simulink model "SF004B_AssiSumLim"  (R2013b)
settings: Solver=FixedStepDiscrete  StartTime=0.0  StopTime=1  FixedStep=.002  RelTol=1e-3
values from neighbouring files (symbols this model uses):
  AssiSumLimNtc0x0C4FailStep = DataDict.Calibration    [SF004B_AssiSumLim_DataDict.m]
  AssiSumLimNtc0x0C4PassStep = DataDict.Calibration    [SF004B_AssiSumLim_DataDict.m]
  AssiSumLimPullCmpLim = DataDict.Calibration    [SF004B_AssiSumLim_DataDict.m]
  CMDTHD_MOTNWTMTR_F32 = DataDict.Constant    [SF004B_AssiSumLim_DataDict.m]
  E_NOT_OK = DataDict.Constant    [AR200A_ArSuprt_DataDict.m]
  E_OK = DataDict.Constant    [AR200A_ArSuprt_DataDict.m]
  MOTTQZERO_MOTNWTMTR_F32 = DataDict.Constant    [SF004B_AssiSumLim_DataDict.m]
  VEHSPDTHD_KPH_F32 = DataDict.Constant    [SF004B_AssiSumLim_DataDict.m]
undefined symbols (not defined in the file or in its folder): NtcNr1, NtcSts1, SigQlfr1
libraries: simulink x11, NexteerUtilities x7, NxtrSign x1, NxtrAbslt x1
(part 2 of 3)

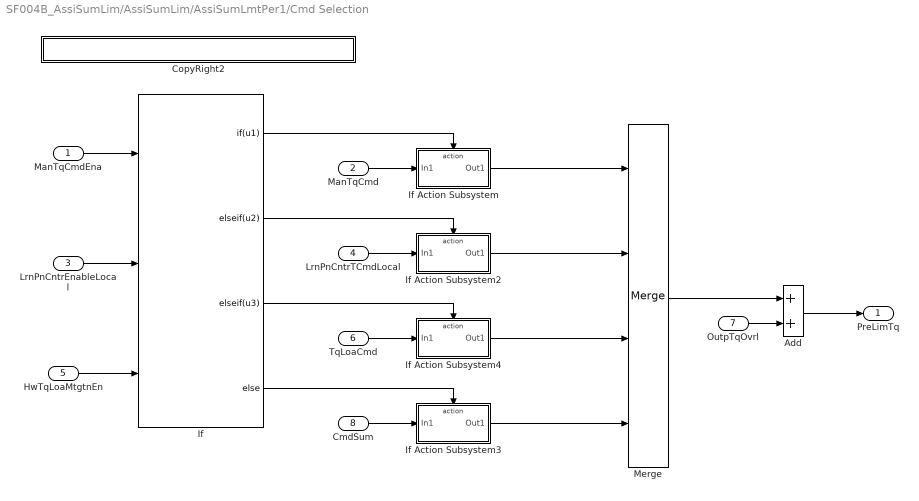
== system SF004B_AssiSumLim/AssiSumLim/AssiSumLmtPer1/Cmd Selection ==
  ManTqCmdEna : Inport  OutDataTypeStr=boolean  PortDimensions=1
  ManTqCmd : Inport  RequirementInfo="{'linktype_rmi_doors' '00007fee (/E-STEER Core/SubSystem Specifications/Application Functions/SF004B Assist Summation and Limiting- Current)' '#SF004B_259' 'true' 'REQ:  SF004B_259' '' } %GIDa_6d4687b5_3845_4db2_a601_45ef4cdee017"  Port=2  PortDimensions=1
  LrnPnCntrEnableLocal : Inport  Port=3  PortDimensions=1
  LrnPnCntrTCmdLocal : Inport  RequirementInfo="{'linktype_rmi_doors' '00007fee (/E-STEER Core/SubSystem Specifications/Application Functions/SF004B Assist Summation and Limiting- Current)' '#SF004B_259' 'true' 'REQ:  SF004B_259' '' } %GIDa_5a22f24a_6e36_40a7_96fa_9b9f9ce3bdd4"  Port=4  PortDimensions=1
  HwTqLoaMtgtnEn : Inport  Port=5  PortDimensions=1
  TqLoaCmd : Inport  RequirementInfo="{'linktype_rmi_doors' '00007fee (/E-STEER Core/SubSystem Specifications/Application Functions/SF004B Assist Summation and Limiting- Current)' '#SF004B_259' 'true' 'REQ:  SF004B_259' '' } %GIDa_d1377691_6c28_435b_bb8c_3dc15aacdf96"  Port=6  PortDimensions=1
  OutpTqOvrl : Inport  RequirementInfo="{'linktype_rmi_doors' '00007fee (/E-STEER Core/SubSystem Specifications/Application Functions/SF004B Assist Summation and Limiting- Current)' '#SF004B_262' 'true' 'REQ:  SF004B_262' '' } %GIDa_e8533355_9a04_466e_861e_ebd78117bea2"  Port=7
  CmdSum : Inport  RequirementInfo="{'linktype_rmi_doors' '00007fee (/E-STEER Core/SubSystem Specifications/Application Functions/SF004B Assist Summation and Limiting- Current)' '#SF004B_259' 'true' 'REQ:  SF004B_259' '' } %GIDa_7c3c2e40_c5fa_4ce2_b662_add04edc3132"  Port=8
  Add : Sum  RequirementInfo="{'linktype_rmi_doors' '00007fee (/E-STEER Core/SubSystem Specifications/Application Functions/SF004B Assist Summation and Limiting- Current)' '#SF004B_262' 'true' 'REQ:  SF004B_262' '' } %GIDa_34ce2345_5df1_4df2_a470_66ac93518d9f"
  CopyRight2 : Subsystem  Description=|  mask(Copyright Information){none=on}
      | Copyright info block.                                               
      |                                                                     
      | Place copyright information at the top of every subsystem in design.
      mask prompts: none "No parameters"
      mask help: Place copyright information at the top of every subsystem in design.
      mask Display:
      | NxtrConf = 'Nexteer Confidential';
      | 
      | sys = bdroot; %handle for the current model ("system")
      | first = get_param(sys,'Created');
      | first = first(end-3:end);  %year is last four digits
      | 
      | last = get_param(sys,'LastModifiedDate');
      | if isempty(last)
      |     last = datestr(now,'yyyy');
      | else
      |     last = last(end-3:end);
      | end
      | 
      | if strcmp(first,last)
      |     fprintf('%s -- Copyright %s Nexteer',NxtrConf,first)
      | else
      |     fprintf('%s -- %s%s- %s Nexteer',NxtrConf,char(169),first,last)
      | end
  If : If  RequirementInfo="{'linktype_rmi_doors' '00007fee (/E-STEER Core/SubSystem Specifications/Application Functions/SF004B Assist Summation and Limiting- Current)' '#SF004B_219' 'true' 'REQ:  SF004B_219' '' } %GIDa_35ee30c3_2e73_4baf_af04_8a15c809cf7f"  NumInputs=3  IfExpression=u1  ElseIfExpressions=u2, u3
  If Action Subsystem : Subsystem  TreatAsAtomicUnit=on
      settings: RTWSystemCode=Inline
  If Action Subsystem2 : Subsystem  TreatAsAtomicUnit=on
      settings: RTWSystemCode=Inline
  If Action Subsystem3 : Subsystem  TreatAsAtomicUnit=on
      settings: RTWSystemCode=Inline
  If Action Subsystem4 : Subsystem  TreatAsAtomicUnit=on
      settings: RTWSystemCode=Inline
  Merge : Merge  Inputs=4
  PreLimTq : Outport
  wires:
  Merge/1 -> Add/1
  ManTqCmd/1 -> If Action Subsystem/1(In1)
  LrnPnCntrTCmdLocal/1 -> If Action Subsystem2/1(In1)
  TqLoaCmd/1 -> If Action Subsystem4/1(In1)
  CmdSum/1 -> If Action Subsystem3/1(In1)
  If/1 -> If Action Subsystem/Action
  If/2 -> If Action Subsystem2/Action
  If/3 -> If Action Subsystem4/Action
  If/4 -> If Action Subsystem3/Action
  ManTqCmdEna/1 -> If/1
  LrnPnCntrEnableLocal/1 -> If/2
  HwTqLoaMtgtnEn/1 -> If/3
  If Action Subsystem2/1(Out1) -> Merge/2
  If Action Subsystem/1(Out1) -> Merge/1
  If Action Subsystem4/1(Out1) -> Merge/3
  If Action Subsystem3/1(Out1) -> Merge/4
  OutpTqOvrl/1 -> Add/2
  Add/1 -> PreLimTq/1

== system SF004B_AssiSumLim/AssiSumLim/AssiSumLmtPer1/Cmd Summation ==
  AssiCmd : Inport  PortDimensions=1
  EotAssiSca : Inport  Port=2  PortDimensions=1
  LimdRtn : Inport  Port=3  PortDimensions=1
  CombdDampg : Inport  Port=4  PortDimensions=1
  AssisEotDampg : Inport  Port=5  PortDimensions=1
  WhlImbRejctnCmd : Inport  Port=6  PortDimensions=1
  PullCmpCmd : Inport  RequirementInfo={} %GIDa_3c33220d_3b7c_4bff_a881_a0220ab0f687  Port=7
  TqSteerMtgtnCmd : Inport  RequirementInfo={} %GIDa_a55a9c38_6f5b_4402_afc7_80609bbfcfbd  Port=8
  EotActvCmd : Inport  Port=9  PortDimensions=1
  CopyRight2 : Subsystem  Description=|  mask(Copyright Information){none=on}
      | Copyright info block.                                               
      |                                                                     
      | Place copyright information at the top of every subsystem in design.
      mask prompts: none "No parameters"
      mask help: Place copyright information at the top of every subsystem in design.
      mask Display:
      | NxtrConf = 'Nexteer Confidential';
      | 
      | sys = bdroot; %handle for the current model ("system")
      | first = get_param(sys,'Created');
      | first = first(end-3:end);  %year is last four digits
      | 
      | last = get_param(sys,'LastModifiedDate');
      | if isempty(last)
      |     last = datestr(now,'yyyy');
      | else
      |     last = last(end-3:end);
      | end
      | 
      | if strcmp(first,last)
      |     fprintf('%s -- Copyright %s Nexteer',NxtrConf,first)
      | else
      |     fprintf('%s -- %s%s- %s Nexteer',NxtrConf,char(169),first,last)
      | end
  Product : Product  RequirementInfo="{'linktype_rmi_doors' '00007fee (/E-STEER Core/SubSystem Specifications/Application Functions/SF004B Assist Summation and Limiting- Current)' '#SF004B_213' 'true' 'REQ:  SF004B_213' '' } %GIDa_54f00f48_10ff_4ca6_98ab_f17879de9b5f"  RndMeth=Zero
  Summation : Sum  RequirementInfo="{'linktype_rmi_doors' '00007fee (/E-STEER Core/SubSystem Specifications/Application Functions/SF004B Assist Summation and Limiting- Current)' '#SF004B_216' 'true' 'REQ:  SF004B_216' '' } %GIDa_b057e6a3_dc30_4611_b70e_8624ca67ab72"  Inputs=+---++++
  CmdSum : Outport
  wires:
  Summation/1 -> CmdSum/1
  EotAssiSca/1 -> Product/2
  AssiCmd/1 -> Product/1
  CombdDampg/1 -> Summation/3
  LimdRtn/1 -> Summation/2
  Product/1 -> Summation/1  "ScaldAssiCmd"
  AssisEotDampg/1 -> Summation/4
  WhlImbRejctnCmd/1 -> Summation/5
  TqSteerMtgtnCmd/1 -> Summation/6
  EotActvCmd/1 -> Summation/8
  PullCmpCmd/1 -> Summation/7

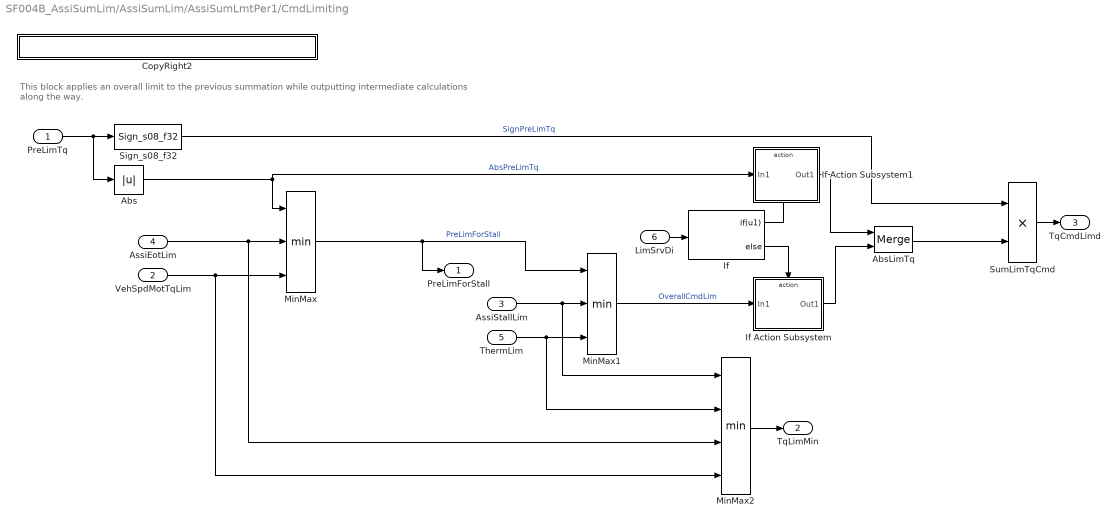
== system SF004B_AssiSumLim/AssiSumLim/AssiSumLmtPer1/CmdLimiting ==
  note: This block applies an overall limit to the previous summation while outputting intermediate calculations along the way.
  PreLimTq : Inport
  VehSpdMotTqLim : Inport  Port=2
  AssiStallLim : Inport  Port=3
  AssiEotLim : Inport  Port=4
  ThermLim : Inport  Port=5
  LimSrvDi : Inport  RequirementInfo={} %GIDa_99432472_4a71_4873_a7a5_b3a83e1be238  Port=6
  Abs : Abs
  AbsLimTq : Merge
  CopyRight2 : Subsystem  Description=|  mask(Copyright Information){none=on}
      | Copyright info block.                                               
      |                                                                     
      | Place copyright information at the top of every subsystem in design.
      mask prompts: none "No parameters"
      mask help: Place copyright information at the top of every subsystem in design.
      mask Display:
      | NxtrConf = 'Nexteer Confidential';
      | 
      | sys = bdroot; %handle for the current model ("system")
      | first = get_param(sys,'Created');
      | first = first(end-3:end);  %year is last four digits
      | 
      | last = get_param(sys,'LastModifiedDate');
      | if isempty(last)
      |     last = datestr(now,'yyyy');
      | else
      |     last = last(end-3:end);
      | end
      | 
      | if strcmp(first,last)
      |     fprintf('%s -- Copyright %s Nexteer',NxtrConf,first)
      | else
      |     fprintf('%s -- %s%s- %s Nexteer',NxtrConf,char(169),first,last)
      | end
  If : If  RequirementInfo="{'linktype_rmi_doors' '00007fee (/E-STEER Core/SubSystem Specifications/Application Functions/SF004B Assist Summation and Limiting- Current)' '#SF004B_274' 'true' 'REQ:  SF004B_274' '' ; 'linktype_rmi_doors' '00007fee (/E-STEER Core/SubSystem Specifications/Application Functions/SF004B Assist Summation and Limiting- Current)' '#SF004B_231' 'true' 'REQ:  SF004B_231' '' } %GIDa_b6ca4058_5217_4cfe_92e9_f2747dcd1412"  IfExpression=u1
  If Action Subsystem : Subsystem  TreatAsAtomicUnit=on
  If Action Subsystem1 : Subsystem  TreatAsAtomicUnit=on
  MinMax : MinMax  RequirementInfo="{'linktype_rmi_doors' '00007fee (/E-STEER Core/SubSystem Specifications/Application Functions/SF004B Assist Summation and Limiting- Current)' '#SF004B_233' 'true' 'REQ:  SF004B_233' '' } %GIDa_b7889423_6edb_4d87_96b6_21fb77770748"  Inputs=3
  MinMax1 : MinMax  RequirementInfo="{'linktype_rmi_doors' '00007fee (/E-STEER Core/SubSystem Specifications/Application Functions/SF004B Assist Summation and Limiting- Current)' '#SF004B_232' 'true' 'REQ:  SF004B_232' '' } %GIDa_f7d227db_8738_4fd0_b4dd_de7410152b8b"  Inputs=3
  MinMax2 : MinMax  RequirementInfo="{'linktype_rmi_doors' '00007fee (/E-STEER Core/SubSystem Specifications/Application Functions/SF004B Assist Summation and Limiting- Current)' '#SF004B_234' 'true' 'REQ:  SF004B_234' '' } %GIDa_87d08d71_c97c_4c6d_9ff2_320bb954175b"  Inputs=4
  Sign_s08_f32 : NxtrSign/Sign_s08_f32  SFunctionSpec=int8 y1 = Sign_s08_f32(single u1)
  SumLimTqCmd : Product  RequirementInfo={} %GIDa_2c601304_2811_4536_8544_69d3b3eae512  RndMeth=Zero
  PreLimForStall : Outport
  TqLimMin : Outport  Port=2
  TqCmdLimd : Outport  Port=3
  wires:
  PreLimTq/1 -> Abs/1, Sign_s08_f32/1
  AssiEotLim/1 -> MinMax2/3, MinMax/2
  Abs/1 -> If Action Subsystem1/1(In1), MinMax/1  "AbsPreLimTq"
  MinMax1/1 -> If Action Subsystem/1(In1)  "OverallCmdLim"
  LimSrvDi/1 -> If/1
  VehSpdMotTqLim/1 -> MinMax2/4, MinMax/3
  AssiStallLim/1 -> MinMax2/1, MinMax1/2
  ThermLim/1 -> MinMax2/2, MinMax1/3
  MinMax/1 -> MinMax1/1, PreLimForStall/1  "PreLimForStall"
  AbsLimTq/1 -> SumLimTqCmd/2
  Sign_s08_f32/1 -> SumLimTqCmd/1  "SignPreLimTq"
  SumLimTqCmd/1 -> TqCmdLimd/1
  MinMax2/1 -> TqLimMin/1
  If/1 -> If Action Subsystem1/Action
  If/2 -> If Action Subsystem/Action
  If Action Subsystem1/1(Out1) -> AbsLimTq/1
  If Action Subsystem/1(Out1) -> AbsLimTq/2

== system SF004B_AssiSumLim/AssiSumLim/AssiSumLmtPer1/CopyRight2 ==

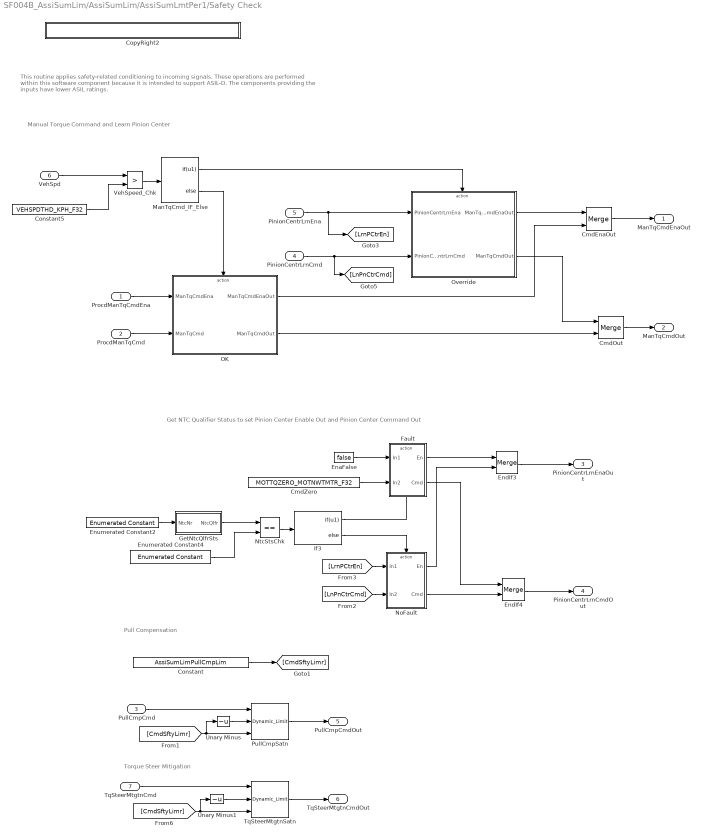
== system SF004B_AssiSumLim/AssiSumLim/AssiSumLmtPer1/Safety Check ==
  note: Get NTC Qualifier Status to set Pinion Center Enable Out and Pinion Center Command Out
  note: This routine applies safety-related conditioning to incoming signals.  These operations are performed within this software component
      | because it is intended to support ASIL-D.  The components providing the inputs have lower ASIL ratings.
  note: Pull Compensation
  note: Manual Torque Command and Learn Pinion Center
  note: Torque Steer Mitigation
  ProcdManTqCmdEna : Inport  OutDataTypeStr=boolean  PortDimensions=1
  ProcdManTqCmd : Inport  Port=2  PortDimensions=1
  PullCmpCmd : Inport  Port=3  PortDimensions=1
  PinionCentrLrnCmd : Inport  Port=4  PortDimensions=1
  PinionCentrLrnEna : Inport  Port=5  PortDimensions=1
  VehSpd : Inport  RequirementInfo="{'linktype_rmi_doors' '00007fee (/E-STEER Core/SubSystem Specifications/Application Functions/SF004B Assist Summation and Limiting- Current)' '#SF004B_290' 'true' 'REQ:  SF004B_290' '' ; 'linktype_rmi_doors' '00007fee (/E-STEER Core/SubSystem Specifications/Application Functions/SF004B Assist Summation and Limiting- Current)' '#SF004B_291' 'true' 'REQ:  SF004B_291' '' } %GIDa_9e2345ee_1316_4978_91a9_3c7026d77478"  Port=6  PortDimensions=1
  TqSteerMtgtnCmd : Inport  Port=7  PortDimensions=1
  CmdEnaOut : Merge
  CmdOut : Merge
  CmdZero : Constant  RequirementInfo="{'linktype_rmi_doors' '00007fee (/E-STEER Core/SubSystem Specifications/Application Functions/SF004B Assist Summation and Limiting- Current)' '#SF004B_273' 'true' 'REQ:  SF004B_273' '' } %GIDa_72c80312_63d9_41e1_a105_02d9b74c32c9"  Value=MOTTQZERO_MOTNWTMTR_F32
  Constant : Constant  RequirementInfo="{'linktype_rmi_doors' '00007fee (/E-STEER Core/SubSystem Specifications/Application Functions/SF004B Assist Summation and Limiting- Current)' '#SF004B_212' 'true' 'REQ:  SF004B_212' '' ; 'linktype_rmi_doors' '00007fee (/E-STEER Core/SubSystem Specifications/Application Functions/SF004B Assist Summation and Limiting- Current)' '#SF004B_296' 'true' 'REQ:  SF004B_296' '' } %GIDa_3116ad40_ee56_4034_a9ad_0e11ebed5c7d"  Value=AssiSumLimPullCmpLim
  Constant5 : Constant  RequirementInfo="{'linktype_rmi_doors' '00007fee (/E-STEER Core/SubSystem Specifications/Application Functions/SF004B Assist Summation and Limiting- Current)' '#SF004B_290' 'true' 'REQ:  SF004B_290' '' ; 'linktype_rmi_doors' '00007fee (/E-STEER Core/SubSystem Specifications/Application Functions/SF004B Assist Summation and Limiting- Current)' '#SF004B_291' 'true' 'REQ:  SF004B_291' '' } %GIDa_d7f1dc31_adb8_4977_a360_33e586f4483f"  Value=VEHSPDTHD_KPH_F32
  CopyRight2 : Subsystem  Description=|  mask(Copyright Information){none=on}
      | Copyright info block.                                               
      |                                                                     
      | Place copyright information at the top of every subsystem in design.
      mask prompts: none "No parameters"
      mask help: Place copyright information at the top of every subsystem in design.
      mask Display:
      | NxtrConf = 'Nexteer Confidential';
      | 
      | sys = bdroot; %handle for the current model ("system")
      | first = get_param(sys,'Created');
      | first = first(end-3:end);  %year is last four digits
      | 
      | last = get_param(sys,'LastModifiedDate');
      | if isempty(last)
      |     last = datestr(now,'yyyy');
      | else
      |     last = last(end-3:end);
      | end
      | 
      | if strcmp(first,last)
      |     fprintf('%s -- Copyright %s Nexteer',NxtrConf,first)
      | else
      |     fprintf('%s -- %s%s- %s Nexteer',NxtrConf,char(169),first,last)
      | end
  EnaFalse : Constant  RequirementInfo="{'linktype_rmi_doors' '00007fee (/E-STEER Core/SubSystem Specifications/Application Functions/SF004B Assist Summation and Limiting- Current)' '#SF004B_272' 'true' 'REQ:  SF004B_272' '' } %GIDa_5ff0557c_fca9_4b53_a4d3_a49375b62df5"  Value=false  OutDataTypeStr=boolean
  EndIf3 : Merge
  EndIf4 : Merge
  Enumerated Constant2 : simulink/Sources/Enumerated Constant  RequirementInfo="{'linktype_rmi_doors' '00007fee (/E-STEER Core/SubSystem Specifications/Application Functions/SF004B Assist Summation and Limiting- Current)' '#SF004B_270' 'true' 'REQ:  SF004B_270' '' } %GIDa_fe97f3de_4aa7_4587_b943_1a0b68072b4c"  OutDataTypeStr=Enum: NtcNr1  Value=NtcNr1.NTCNR_0X0C4  SampleTime=inf
  Enumerated Constant4 : simulink/Sources/Enumerated Constant  RequirementInfo="{'linktype_rmi_doors' '00007fee (/E-STEER Core/SubSystem Specifications/Application Functions/SF004B Assist Summation and Limiting- Current)' '#SF004B_270' 'true' 'REQ:  SF004B_270' '' } %GIDa_63663681_ffa3_4a91_a470_a2544b7c0835"  OutDataTypeStr=Enum: SigQlfr1  Value=SigQlfr1.SIGQLFR_FAILD  SampleTime=inf
  Fault : Subsystem  RequirementInfo="{'linktype_rmi_doors' '00007fee (/E-STEER Core/SubSystem Specifications/Application Functions/SF004B Assist Summation and Limiting- Current)' '#SF004B_270' 'true' 'REQ:  SF004B_270' '' } %GIDa_a6ae2e68_5cf5_45c1_b47e_16fabd600c68"  TreatAsAtomicUnit=on
      settings: RTWSystemCode=Inline
  GetNtcQlfrSts : Subsystem  RequirementInfo="{'linktype_rmi_doors' '00007fee (/E-STEER Core/SubSystem Specifications/Application Functions/SF004B Assist Summation and Limiting- Current)' '#SF004B_270' 'true' 'REQ:  SF004B_270' '' } %GIDa_160041d5_3f9d_403a_ac84_d13c70ea3b97"  TreatAsAtomicUnit=on  mask(GetNTC){}
      mask help: GetNTC library block
      settings: RTWSystemCode=Inline
  If3 : If  RequirementInfo="{'linktype_rmi_doors' '00007fee (/E-STEER Core/SubSystem Specifications/Application Functions/SF004B Assist Summation and Limiting- Current)' '#SF004B_270' 'true' 'REQ:  SF004B_270' '' } %GIDa_dbf14775_42f2_44d6_bdcc_28cea20182c7"  IfExpression=u1
  ManTqCmd_IF_Else : If  RequirementInfo="{'linktype_rmi_doors' '00007fee (/E-STEER Core/SubSystem Specifications/Application Functions/SF004B Assist Summation and Limiting- Current)' '#SF004B_290' 'true' 'REQ:  SF004B_290' '' ; 'linktype_rmi_doors' '00007fee (/E-STEER Core/SubSystem Specifications/Application Functions/SF004B Assist Summation and Limiting- Current)' '#SF004B_291' 'true' 'REQ:  SF004B_291' '' } %GIDa_5ecbdf41_6b0b_44e6_abca_066fe4f2cb92"  IfExpression=u1
  NoFault : Subsystem  TreatAsAtomicUnit=on
      settings: RTWSystemCode=Inline
  NtcStsChk : RelationalOperator  RequirementInfo="{'linktype_rmi_doors' '00007fee (/E-STEER Core/SubSystem Specifications/Application Functions/SF004B Assist Summation and Limiting- Current)' '#SF004B_270' 'true' 'REQ:  SF004B_270' '' } %GIDa_0dad4e9e_7eac_4b84_8c05_cc315494a582"  Operator===  OutDataTypeStr=boolean
  OK : Subsystem  TreatAsAtomicUnit=on
      settings: RTWSystemCode=Inline
  Override : Subsystem  RequirementInfo="{}  %GIDa_68c2586b_0b52_4b35_9c36_d935d27471ff"  TreatAsAtomicUnit=on
      settings: RTWSystemCode=Inline
  PullCmpSatn : NexteerUtilities/Dynamic_Limit  RequirementInfo="{'linktype_rmi_doors' '00007fee (/E-STEER Core/SubSystem Specifications/Application Functions/SF004B Assist Summation and Limiting- Current)' '#SF004B_212' 'true' 'REQ:  SF004B_212' '' } %GIDa_833cf9fb_40c9_409d_b2cf_b906ba45bd8b"
  TqSteerMtgtnSatn : NexteerUtilities/Dynamic_Limit  RequirementInfo="{'linktype_rmi_doors' '00007fee (/E-STEER Core/SubSystem Specifications/Application Functions/SF004B Assist Summation and Limiting- Current)' '#SF004B_296' 'true' 'REQ:  SF004B_296' '' } %GIDa_ee85d5d2_228e_4ce6_90fb_edd95af945f9"
  Unary Minus : UnaryMinus
  Unary Minus1 : UnaryMinus
  VehSpeed_Chk : RelationalOperator  RequirementInfo="{'linktype_rmi_doors' '00007fee (/E-STEER Core/SubSystem Specifications/Application Functions/SF004B Assist Summation and Limiting- Current)' '#SF004B_290' 'true' 'REQ:  SF004B_290' '' ; 'linktype_rmi_doors' '00007fee (/E-STEER Core/SubSystem Specifications/Application Functions/SF004B Assist Summation and Limiting- Current)' '#SF004B_291' 'true' 'REQ:  SF004B_291' '' } %GIDa_a6ce3cb5_8aa4_4683_a921_a710aa676490"  Operator=>  OutDataTypeStr=boolean
  ManTqCmdEnaOut : Outport
  ManTqCmdOut : Outport  Port=2
  PinionCentrLrnEnaOut : Outport  Port=3
  PinionCentrLrnCmdOut : Outport  Port=4
  PullCmpCmdOut : Outport  Port=5
  TqSteerMtgtnCmdOut : Outport  Port=6
  wires:
  PullCmpCmd/1 -> PullCmpSatn/1
  [CmdSftyLimr] -> Unary Minus/1, PullCmpSatn/3
  Unary Minus/1 -> PullCmpSatn/2
  PullCmpSatn/1 -> PullCmpCmdOut/1
  Constant5/1 -> VehSpeed_Chk/2
  TqSteerMtgtnCmd/1 -> TqSteerMtgtnSatn/1
  [CmdSftyLimr] -> Unary Minus1/1, TqSteerMtgtnSatn/3
  Unary Minus1/1 -> TqSteerMtgtnSatn/2
  TqSteerMtgtnSatn/1 -> TqSteerMtgtnCmdOut/1
  Constant/1 -> [CmdSftyLimr]
  VehSpd/1 -> VehSpeed_Chk/1
  VehSpeed_Chk/1 -> ManTqCmd_IF_Else/1
  ManTqCmd_IF_Else/1 -> Override/Action
  ManTqCmd_IF_Else/2 -> OK/Action
  PinionCentrLrnEna/1 -> Override/1(PinionCentrLrnEna), [LrnPCtrEn]
  PinionCentrLrnCmd/1 -> Override/2(PinionCentrLrnCmd), [LnPnCtrCmd]
  ProcdManTqCmdEna/1 -> OK/1(ManTqCmdEna)
  ProcdManTqCmd/1 -> OK/2(ManTqCmd)
  OK/1(ManTqCmdEnaOut) -> CmdEnaOut/2
  Override/2(ManTqCmdOut) -> CmdOut/1
  OK/2(ManTqCmdOut) -> CmdOut/2
  CmdOut/1 -> ManTqCmdOut/1
  If3/1 -> Fault/Action
  EnaFalse/1 -> Fault/1(In1)
  If3/2 -> NoFault/Action
  CmdZero/1 -> Fault/2(In2)
  Fault/1(En) -> EndIf3/1
  NoFault/1(En) -> EndIf3/2
  Fault/2(Cmd) -> EndIf4/1
  NoFault/2(Cmd) -> EndIf4/2
  EndIf3/1 -> PinionCentrLrnEnaOut/1
  [LnPnCtrCmd] -> NoFault/2(In2)
  [LrnPCtrEn] -> NoFault/1(In1)
  Enumerated Constant2/1 -> GetNtcQlfrSts/1(NtcNr)
  GetNtcQlfrSts/1(NtcQlfr) -> NtcStsChk/1
  Enumerated Constant4/1 -> NtcStsChk/2
  NtcStsChk/1 -> If3/1
  Override/1(ManTqCmdEnaOut) -> CmdEnaOut/1
  CmdEnaOut/1 -> ManTqCmdEnaOut/1
  EndIf4/1 -> PinionCentrLrnCmdOut/1

== system SF004B_AssiSumLim/AssiSumLim/SetManTqCmd/CopyRight2 ==

== system SF004B_AssiSumLim/AssiSumLim/SetManTqCmd/ELSE ==
  In1 : Inport
  In2 : Inport  Port=2
  In3 : Inport  Port=3
  Action Port : ActionPort  ActionType=else
  CopyRight2 : Subsystem  Description=|  mask(Copyright Information){none=on}
      | Copyright info block.                                               
      |                                                                     
      | Place copyright information at the top of every subsystem in design.
      mask prompts: none "No parameters"
      mask help: Place copyright information at the top of every subsystem in design.
      mask Display:
      | NxtrConf = 'Nexteer Confidential';
      | 
      | sys = bdroot; %handle for the current model ("system")
      | first = get_param(sys,'Created');
      | first = first(end-3:end);  %year is last four digits
      | 
      | last = get_param(sys,'LastModifiedDate');
      | if isempty(last)
      |     last = datestr(now,'yyyy');
      | else
      |     last = last(end-3:end);
      | end
      | 
      | if strcmp(first,last)
      |     fprintf('%s -- Copyright %s Nexteer',NxtrConf,first)
      | else
      |     fprintf('%s -- %s%s- %s Nexteer',NxtrConf,char(169),first,last)
      | end
  Out1 : Outport
  Out2 : Outport  Port=2
  Out3 : Outport  Port=3
  wires:
  In3/1 -> Out3/1
  In2/1 -> Out2/1
  In1/1 -> Out1/1

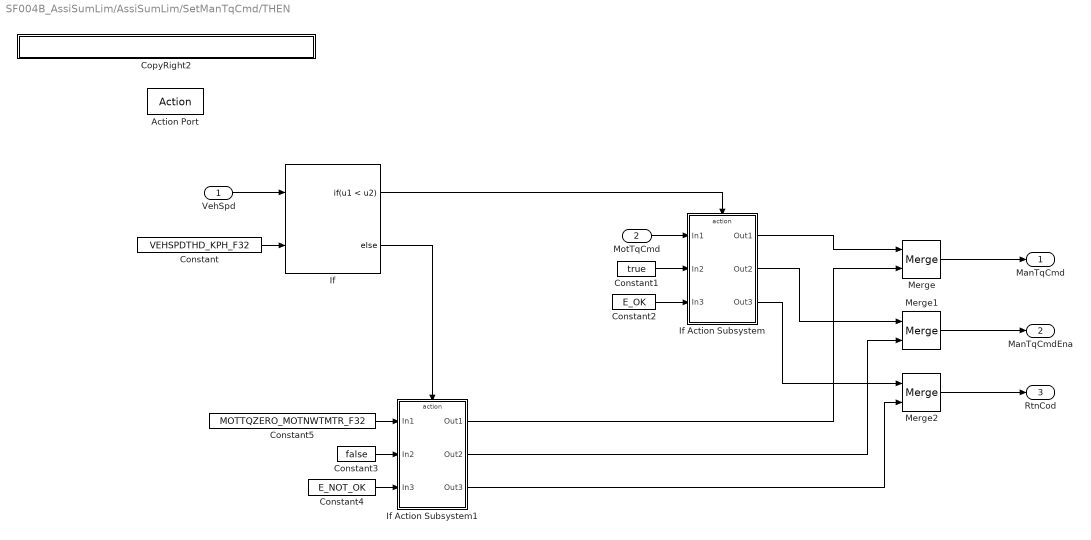
== system SF004B_AssiSumLim/AssiSumLim/SetManTqCmd/THEN ==
  VehSpd : Inport
  MotTqCmd : Inport  RequirementInfo="{'linktype_rmi_doors' '00007fee (/E-STEER Core/SubSystem Specifications/Application Functions/SF004B Assist Summation and Limiting- Current)' '#SF004B_285' 'true' 'REQ:  SF004B_285' '' } %GIDa_ad554846_ed1e_4125_b073_215b713db520"  Port=2
  Action Port : ActionPort  ActionType=then
  Constant : Constant  RequirementInfo="{'linktype_rmi_doors' '00007fee (/E-STEER Core/SubSystem Specifications/Application Functions/SF004B Assist Summation and Limiting- Current)' '#SF004B_285' 'true' 'REQ:  SF004B_285' '' ; 'linktype_rmi_doors' '00007fee (/E-STEER Core/SubSystem Specifications/Application Functions/SF004B Assist Summation and Limiting- Current)' '#SF004B_286' 'true' 'REQ:  SF004B_286' '' } %GIDa_a3485ce7_cedc_4d08_b240_e20550bef289"  Value=VEHSPDTHD_KPH_F32
  Constant1 : Constant  RequirementInfo="{'linktype_rmi_doors' '00007fee (/E-STEER Core/SubSystem Specifications/Application Functions/SF004B Assist Summation and Limiting- Current)' '#SF004B_285' 'true' 'REQ:  SF004B_285' '' } %GIDa_377e025c_757b_4bb0_b1c8_47e28a623a60"  Value=true
  Constant2 : Constant  Value=E_OK
  Constant3 : Constant  RequirementInfo="{'linktype_rmi_doors' '00007fee (/E-STEER Core/SubSystem Specifications/Application Functions/SF004B Assist Summation and Limiting- Current)' '#SF004B_286' 'true' 'REQ:  SF004B_286' '' } %GIDa_d6cba000_ab46_4a38_9acb_d238c8928b85"  Value=false
  Constant4 : Constant  Value=E_NOT_OK
  Constant5 : Constant  RequirementInfo="{'linktype_rmi_doors' '00007fee (/E-STEER Core/SubSystem Specifications/Application Functions/SF004B Assist Summation and Limiting- Current)' '#SF004B_286' 'true' 'REQ:  SF004B_286' '' } %GIDa_7a4ed781_fc7c_4c5a_ba35_53cc324903c0"  Value=MOTTQZERO_MOTNWTMTR_F32
  CopyRight2 : Subsystem  Description=|  mask(Copyright Information){none=on}
      | Copyright info block.                                               
      |                                                                     
      | Place copyright information at the top of every subsystem in design.
      mask prompts: none "No parameters"
      mask help: Place copyright information at the top of every subsystem in design.
      mask Display:
      | NxtrConf = 'Nexteer Confidential';
      | 
      | sys = bdroot; %handle for the current model ("system")
      | first = get_param(sys,'Created');
      | first = first(end-3:end);  %year is last four digits
      | 
      | last = get_param(sys,'LastModifiedDate');
      | if isempty(last)
      |     last = datestr(now,'yyyy');
      | else
      |     last = last(end-3:end);
      | end
      | 
      | if strcmp(first,last)
      |     fprintf('%s -- Copyright %s Nexteer',NxtrConf,first)
      | else
      |     fprintf('%s -- %s%s- %s Nexteer',NxtrConf,char(169),first,last)
      | end
  If : If  RequirementInfo="{'linktype_rmi_doors' '00007fee (/E-STEER Core/SubSystem Specifications/Application Functions/SF004B Assist Summation and Limiting- Current)' '#SF004B_285' 'true' 'REQ:  SF004B_285' '' ; 'linktype_rmi_doors' '00007fee (/E-STEER Core/SubSystem Specifications/Application Functions/SF004B Assist Summation and Limiting- Current)' '#SF004B_286' 'true' 'REQ:  SF004B_286' '' } %GIDa_47bc5765_27cf_49e3_a3af_b244c05be68c"  NumInputs=2  IfExpression=u1 < u2
  If Action Subsystem : Subsystem  RequirementInfo="{'linktype_rmi_doors' '00007fee (/E-STEER Core/SubSystem Specifications/Application Functions/SF004B Assist Summation and Limiting- Current)' '#SF004B_285' 'true' 'REQ:  SF004B_285' '' } %GIDa_a5140ed2_25d6_4804_98a9_ef8f8d8d2706"  TreatAsAtomicUnit=on
      settings: RTWSystemCode=Inline
  If Action Subsystem1 : Subsystem  RequirementInfo="{'linktype_rmi_doors' '00007fee (/E-STEER Core/SubSystem Specifications/Application Functions/SF004B Assist Summation and Limiting- Current)' '#SF004B_286' 'true' 'REQ:  SF004B_286' '' } %GIDa_5baa54f2_0d06_40cd_afad_7039258b1393"  TreatAsAtomicUnit=on
      settings: RTWSystemCode=Inline
  Merge : Merge
  Merge1 : Merge
  Merge2 : Merge
  ManTqCmd : Outport
  ManTqCmdEna : Outport  Port=2
  RtnCod : Outport  Port=3
  wires:
  VehSpd/1 -> If/1
  Constant/1 -> If/2
  MotTqCmd/1 -> If Action Subsystem/1(In1)
  Constant1/1 -> If Action Subsystem/2(In2)
  Constant2/1 -> If Action Subsystem/3(In3)
  If/1 -> If Action Subsystem/Action
  If/2 -> If Action Subsystem1/Action
  Constant5/1 -> If Action Subsystem1/1(In1)
  Constant3/1 -> If Action Subsystem1/2(In2)
  Constant4/1 -> If Action Subsystem1/3(In3)
  Merge/1 -> ManTqCmd/1
  Merge1/1 -> ManTqCmdEna/1
  Merge2/1 -> RtnCod/1
  If Action Subsystem/1(Out1) -> Merge/1
  If Action Subsystem1/1(Out1) -> Merge/2
  If Action Subsystem/2(Out2) -> Merge1/1
  If Action Subsystem1/2(Out2) -> Merge1/2
  If Action Subsystem/3(Out3) -> Merge2/1
  If Action Subsystem1/3(Out3) -> Merge2/2

== system SF004B_AssiSumLim/ISO Fault Debounce/DiagMgr/CopyRight2 ==

== system SF004B_AssiSumLim/ISO Fault Debounce/DiagMgr/If Action Subsystem ==
  EA : Inport
  Qlf : Inport  Port=2
  Action Port : ActionPort  ActionType=else
  EAo : Outport
  Qlfo : Outport  Port=2
  wires:
  EA/1 -> EAo/1
  Qlf/1 -> Qlfo/1

== system SF004B_AssiSumLim/ISO Fault Debounce/DiagMgr/If Action Subsystem1 ==
  Qlf : Inport
  EA : Inport  Port=2
  Action Port : ActionPort  ActionType=then
  Qlfo : Outport
  EAo : Outport  Port=2
  wires:
  EA/1 -> EAo/1
  Qlf/1 -> Qlfo/1

== system SF004B_AssiSumLim/ISO Fault Debounce/DiagMgr/If Action Subsystem3 ==
  In1 : Inport
  Action Port : ActionPort  ActionType=then
  Out1 : Outport
  wires:
  In1/1 -> Out1/1

== system SF004B_AssiSumLim/ISO Fault Debounce/DiagMgr/If Action Subsystem4 ==
  In1 : Inport
  Action Port : ActionPort  ActionType=else
  Out1 : Outport
  wires:
  In1/1 -> Out1/1

== system SF004B_AssiSumLim/ISO Fault Debounce/DiagMgr/NTCSTS_FAILD ==
  EA : Inport
  Qlf : Inport  Port=2
  Action Port : ActionPort  ActionType=case
  EAo : Outport
  Qlfo : Outport  Port=2
  wires:
  EA/1 -> EAo/1
  Qlf/1 -> Qlfo/1

== system SF004B_AssiSumLim/ISO Fault Debounce/DiagMgr/NTCSTS_PASSD ==
  EA : Inport
  Qlf : Inport  Port=2
  Action Port : ActionPort  ActionType=case
  EAo : Outport
  Qlfo : Outport  Port=2
  wires:
  EA/1 -> EAo/1
  Qlf/1 -> Qlfo/1

== system SF004B_AssiSumLim/ISO Fault Debounce/DiagMgr/NTCSTS_PREFAILD ==
  EA : Inport
  DS : Inport  Port=2
  TS : Inport  Port=3
  Qlf : Inport  Port=4
  Action Port : ActionPort  ActionType=case
  CopyRight2 : Subsystem  Description=|  mask(Copyright Information){none=on}
      | Copyright info block.                                               
      |                                                                     
      | Place copyright information at the top of every subsystem in design.
      mask prompts: none "No parameters"
      mask help: Place copyright information at the top of every subsystem in design.
      mask Display:
      | NxtrConf = 'Nexteer Confidential';
      | 
      | sys = bdroot; %handle for the current model ("system")
      | first = get_param(sys,'Created');
      | first = first(end-3:end);  %year is last four digits
      | 
      | last = get_param(sys,'LastModifiedDate');
      | if isempty(last)
      |     last = datestr(now,'yyyy');
      | else
      |     last = last(end-3:end);
      | end
      | 
      | if strcmp(first,last)
      |     fprintf('%s -- Copyright %s Nexteer',NxtrConf,first)
      | else
      |     fprintf('%s -- %s%s- %s Nexteer',NxtrConf,char(169),first,last)
      | end
  Data Type Conversion : DataTypeConversion
  If : If  IfExpression=u1 <= 0
  If Action Subsystem : Subsystem  TreatAsAtomicUnit=on
  If Action Subsystem1 : Subsystem  TreatAsAtomicUnit=on
  Merge : Merge
  Merge1 : Merge
  EAo : Outport
  Qlfo : Outport  Port=2
  wires:
  EA/1 -> If Action Subsystem1/2(EA), If/1
  If/1 -> If Action Subsystem/Action
  If/2 -> If Action Subsystem1/Action
  DS/1 -> Data Type Conversion/1, If Action Subsystem1/1(DS)
  TS/1 -> If Action Subsystem1/4(TS)
  If Action Subsystem/1(EAo) -> Merge/1
  If Action Subsystem1/1(EAo) -> Merge/2
  If Action Subsystem1/2(Qlfo) -> Merge1/2
  If Action Subsystem/2(Qlfo) -> Merge1/1
  Merge/1 -> EAo/1
  Merge1/1 -> Qlfo/1
  Qlf/1 -> If Action Subsystem/2(Qlf), If Action Subsystem1/3(Qlf)
  Data Type Conversion/1 -> If Action Subsystem/1(DS)

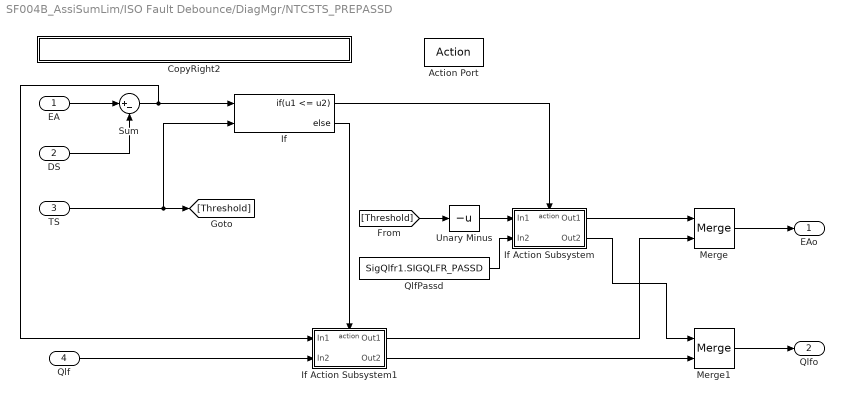
== system SF004B_AssiSumLim/ISO Fault Debounce/DiagMgr/NTCSTS_PREPASSD ==
  EA : Inport
  DS : Inport  Port=2
  TS : Inport  Port=3
  Qlf : Inport  Port=4
  Action Port : ActionPort  ActionType=case
  CopyRight2 : Subsystem  Description=|  mask(Copyright Information){none=on}
      | Copyright info block.                                               
      |                                                                     
      | Place copyright information at the top of every subsystem in design.
      mask prompts: none "No parameters"
      mask help: Place copyright information at the top of every subsystem in design.
      mask Display:
      | NxtrConf = 'Nexteer Confidential';
      | 
      | sys = bdroot; %handle for the current model ("system")
      | first = get_param(sys,'Created');
      | first = first(end-3:end);  %year is last four digits
      | 
      | last = get_param(sys,'LastModifiedDate');
      | if isempty(last)
      |     last = datestr(now,'yyyy');
      | else
      |     last = last(end-3:end);
      | end
      | 
      | if strcmp(first,last)
      |     fprintf('%s -- Copyright %s Nexteer',NxtrConf,first)
      | else
      |     fprintf('%s -- %s%s- %s Nexteer',NxtrConf,char(169),first,last)
      | end
  If : If  NumInputs=2  IfExpression=u1 <= u2
  If Action Subsystem : Subsystem  TreatAsAtomicUnit=on
  If Action Subsystem1 : Subsystem  TreatAsAtomicUnit=on
  Merge : Merge
  Merge1 : Merge
  QlfPassd : Constant  Value=SigQlfr1.SIGQLFR_PASSD  OutDataTypeStr=Enum: SigQlfr1
  Sum : Sum  Inputs=|+-
  Unary Minus : UnaryMinus
  EAo : Outport
  Qlfo : Outport  Port=2
  wires:
  EA/1 -> Sum/1
  DS/1 -> Sum/2
  Sum/1 -> If Action Subsystem1/1(In1), If/1
  TS/1 -> [Threshold], If/2
  If/1 -> If Action Subsystem/Action
  Unary Minus/1 -> If Action Subsystem/1(In1)
  If Action Subsystem/1(Out1) -> Merge/1
  If Action Subsystem1/1(Out1) -> Merge/2
  Merge/1 -> EAo/1
  If Action Subsystem/2(Out2) -> Merge1/1
  If Action Subsystem1/2(Out2) -> Merge1/2
  Merge1/1 -> Qlfo/1
  QlfPassd/1 -> If Action Subsystem/2(In2)
  Qlf/1 -> If Action Subsystem1/2(In2)
  If/2 -> If Action Subsystem1/Action
  [Threshold] -> Unary Minus/1

== system SF004B_AssiSumLim/ISO Fault Debounce/DiagMgr/Set Latch ==
  In1 : Inport
  Action Port : ActionPort  ActionType=then
  Out1 : Outport
  wires:
  In1/1 -> Out1/1

== system SF004B_AssiSumLim/AssiSumLim/AssiSumLmtPer1/Cmd Selection/CopyRight2 ==

== system SF004B_AssiSumLim/AssiSumLim/AssiSumLmtPer1/Cmd Selection/If Action Subsystem ==
  In1 : Inport
  Action Port : ActionPort  ActionType=then
  Out1 : Outport
  wires:
  In1/1 -> Out1/1

== system SF004B_AssiSumLim/AssiSumLim/AssiSumLmtPer1/Cmd Selection/If Action Subsystem2 ==
  In1 : Inport
  Action Port : ActionPort  ActionType=elseif
  Out1 : Outport
  wires:
  In1/1 -> Out1/1

== system SF004B_AssiSumLim/AssiSumLim/AssiSumLmtPer1/Cmd Selection/If Action Subsystem3 ==
  In1 : Inport
  Action Port : ActionPort  ActionType=else
  Out1 : Outport
  wires:
  In1/1 -> Out1/1

== system SF004B_AssiSumLim/AssiSumLim/AssiSumLmtPer1/Cmd Selection/If Action Subsystem4 ==
  In1 : Inport
  Action Port : ActionPort  ActionType=elseif
  Out1 : Outport
  wires:
  In1/1 -> Out1/1

== system SF004B_AssiSumLim/AssiSumLim/AssiSumLmtPer1/Cmd Summation/CopyRight2 ==

== system SF004B_AssiSumLim/AssiSumLim/AssiSumLmtPer1/CmdLimiting/CopyRight2 ==

== system SF004B_AssiSumLim/AssiSumLim/AssiSumLmtPer1/CmdLimiting/If Action Subsystem ==
  In1 : Inport
  Action Port : ActionPort  ActionType=else
  Out1 : Outport
  wires:
  In1/1 -> Out1/1

== system SF004B_AssiSumLim/AssiSumLim/AssiSumLmtPer1/CmdLimiting/If Action Subsystem1 ==
  In1 : Inport
  Action Port : ActionPort  ActionType=then
  Out1 : Outport
  wires:
  In1/1 -> Out1/1

== system SF004B_AssiSumLim/AssiSumLim/AssiSumLmtPer1/Safety Check/CopyRight2 ==

== system SF004B_AssiSumLim/AssiSumLim/AssiSumLmtPer1/Safety Check/Fault ==
  In1 : Inport
  In2 : Inport  Port=2
  Action Port : ActionPort  ActionType=then
  En : Outport
  Cmd : Outport  Port=2
  wires:
  In1/1 -> En/1
  In2/1 -> Cmd/1

== system SF004B_AssiSumLim/AssiSumLim/AssiSumLmtPer1/Safety Check/GetNtcQlfrSts ==
  NtcNr : Inport
  CopyRight2 : Subsystem  Description=|  mask(Copyright Information){none=on}
      | Copyright info block.                                               
      |                                                                     
      | Place copyright information at the top of every subsystem in design.
      mask prompts: none "No parameters"
      mask help: Place copyright information at the top of every subsystem in design.
      mask Display:
      | NxtrConf = 'Nexteer Confidential';
      | 
      | sys = bdroot; %handle for the current model ("system")
      | first = get_param(sys,'Created');
      | first = first(end-3:end);  %year is last four digits
      | 
      | last = get_param(sys,'LastModifiedDate');
      | if isempty(last)
      |     last = datestr(now,'yyyy');
      | else
      |     last = last(end-3:end);
      | end
      | 
      | if strcmp(first,last)
      |     fprintf('%s -- Copyright %s Nexteer',NxtrConf,first)
      | else
      |     fprintf('%s -- %s%s- %s Nexteer',NxtrConf,char(169),first,last)
      | end
  Data Store Read : DataStoreRead  DataStoreName=NtcQlfr
  Terminator : Terminator
  NtcQlfr : Outport
  wires:
  NtcNr/1 -> Terminator/1
  Data Store Read/1 -> NtcQlfr/1

== system SF004B_AssiSumLim/AssiSumLim/AssiSumLmtPer1/Safety Check/NoFault ==
  In1 : Inport
  In2 : Inport  Port=2
  Action Port : ActionPort  ActionType=else
  En : Outport
  Cmd : Outport  Port=2
  wires:
  In1/1 -> En/1
  In2/1 -> Cmd/1

== system SF004B_AssiSumLim/AssiSumLim/AssiSumLmtPer1/Safety Check/OK ==
  note: When vehicle Speed is lesser than thershold, NTC status is set to PREPASSED irrespective of PinionCentrLrnEna and PinionCentrLrnCmd values
  note: When Vehicle Speed is lesser than thershold, pass on Manual Torque Command Enable and Manual Torque Command values
  ManTqCmdEna : Inport  PortDimensions=1
  ManTqCmd : Inport  Port=2  PortDimensions=1
  Action Port : ActionPort  ActionType=else
  Constant5 : Constant  Value=AssiSumLimNtc0x0C4PassStep
  Constant6 : Constant  Value=0
  CopyRight2 : Subsystem  Description=|  mask(Copyright Information){none=on}
      | Copyright info block.                                               
      |                                                                     
      | Place copyright information at the top of every subsystem in design.
      mask prompts: none "No parameters"
      mask help: Place copyright information at the top of every subsystem in design.
      mask Display:
      | NxtrConf = 'Nexteer Confidential';
      | 
      | sys = bdroot; %handle for the current model ("system")
      | first = get_param(sys,'Created');
      | first = first(end-3:end);  %year is last four digits
      | 
      | last = get_param(sys,'LastModifiedDate');
      | if isempty(last)
      |     last = datestr(now,'yyyy');
      | else
      |     last = last(end-3:end);
      | end
      | 
      | if strcmp(first,last)
      |     fprintf('%s -- Copyright %s Nexteer',NxtrConf,first)
      | else
      |     fprintf('%s -- %s%s- %s Nexteer',NxtrConf,char(169),first,last)
      | end
  Enumerated Constant4 : simulink/Sources/Enumerated Constant  OutDataTypeStr=Enum: NtcSts1  Value=NtcSts1.NTCSTS_PREPASSD  SampleTime=inf
  Enumerated Constant6 : simulink/Sources/Enumerated Constant  OutDataTypeStr=Enum: NtcNr1  Value=NtcNr1.NTCNR_0X0C4  SampleTime=inf
  SetNtcSts : Subsystem  mask(SetNTC){}
      mask help: SetNTC library block
  ManTqCmdEnaOut : Outport
  ManTqCmdOut : Outport  Port=2
  wires:
  ManTqCmdEna/1 -> ManTqCmdEnaOut/1
  Enumerated Constant6/1 -> SetNtcSts/1(NtcNr)
  Constant6/1 -> SetNtcSts/2(NtcStInfo)
  Enumerated Constant4/1 -> SetNtcSts/3(NtcSts)
  Constant5/1 -> SetNtcSts/4(DebStep)
  ManTqCmd/1 -> ManTqCmdOut/1

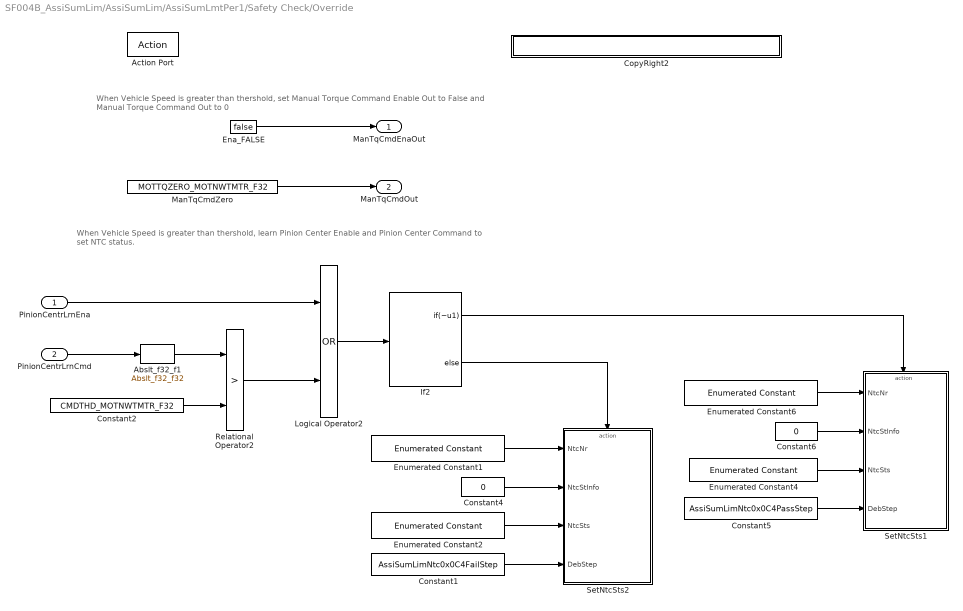
== system SF004B_AssiSumLim/AssiSumLim/AssiSumLmtPer1/Safety Check/Override ==
  note: When Vehicle Speed is greater than thershold, learn Pinion Center Enable and Pinion Center Command to set NTC status.
  note: When Vehicle Speed is greater than thershold, set Manual Torque Command Enable Out to False and Manual Torque Command Out to 0
  PinionCentrLrnEna : Inport  RequirementInfo="{'linktype_rmi_doors' '00007fee (/E-STEER Core/SubSystem Specifications/Application Functions/SF004B Assist Summation and Limiting- Current)' '#SF004B_243' 'true' 'REQ:  SF004B_243' '' } %GIDa_9e4fc770_54e0_43f5_828a_a166ae5fc816"  PortDimensions=1
  PinionCentrLrnCmd : Inport  RequirementInfo="{'linktype_rmi_doors' '00007fee (/E-STEER Core/SubSystem Specifications/Application Functions/SF004B Assist Summation and Limiting- Current)' '#SF004B_243' 'true' 'REQ:  SF004B_243' '' } %GIDa_65ef2a61_f3d0_4c4e_ad4e_9897f68c25f3"  Port=2  PortDimensions=1
  Action Port : ActionPort  ActionType=then
  Abslt_f32_f1 : NxtrAbslt/Abslt_f32_f32  RequirementInfo="{'linktype_rmi_doors' '00007fee (/E-STEER Core/SubSystem Specifications/Application Functions/SF004B Assist Summation and Limiting- Current)' '#SF004B_243' 'true' 'REQ:  SF004B_243' '' } %GIDa_c300bec2_ad78_45a5_a36e_eeda4c320871"  SFunctionSpec=single y1 = Abslt_f32_f32(single u1)
      settings: AttributesFormatString=%<Name>
  Constant1 : Constant  RequirementInfo="{'linktype_rmi_doors' '00007fee (/E-STEER Core/SubSystem Specifications/Application Functions/SF004B Assist Summation and Limiting- Current)' '#SF004B_243' 'true' 'REQ:  SF004B_243' '' } %GIDa_fea1ca1b_0a12_400d_9c37_34f7e49c6fe1"  Value=AssiSumLimNtc0x0C4FailStep
  Constant2 : Constant  RequirementInfo="{'linktype_rmi_doors' '00007fee (/E-STEER Core/SubSystem Specifications/Application Functions/SF004B Assist Summation and Limiting- Current)' '#SF004B_243' 'true' 'REQ:  SF004B_243' '' } %GIDa_bb850e8a_ce3f_4c24_947e_fbea2fdc3179"  Value=CMDTHD_MOTNWTMTR_F32
  Constant4 : Constant  RequirementInfo="{'linktype_rmi_doors' '00007fee (/E-STEER Core/SubSystem Specifications/Application Functions/SF004B Assist Summation and Limiting- Current)' '#SF004B_243' 'true' 'REQ:  SF004B_243' '' } %GIDa_80b57c15_55c8_4063_9c5f_c4a92ca0fd5c"  Value=0
  Constant5 : Constant  RequirementInfo="{'linktype_rmi_doors' '00007fee (/E-STEER Core/SubSystem Specifications/Application Functions/SF004B Assist Summation and Limiting- Current)' '#SF004B_243' 'true' 'REQ:  SF004B_243' '' } %GIDa_857d288b_353f_4557_9e09_a2ed1cb1086d"  Value=AssiSumLimNtc0x0C4PassStep
  Constant6 : Constant  RequirementInfo="{'linktype_rmi_doors' '00007fee (/E-STEER Core/SubSystem Specifications/Application Functions/SF004B Assist Summation and Limiting- Current)' '#SF004B_243' 'true' 'REQ:  SF004B_243' '' } %GIDa_a5f29eaf_ecc8_4c68_b5e1_4727da2de3f0"  Value=0
  CopyRight2 : Subsystem  Description=|  mask(Copyright Information){none=on}
      | Copyright info block.                                               
      |                                                                     
      | Place copyright information at the top of every subsystem in design.
      mask prompts: none "No parameters"
      mask help: Place copyright information at the top of every subsystem in design.
      mask Display:
      | NxtrConf = 'Nexteer Confidential';
      | 
      | sys = bdroot; %handle for the current model ("system")
      | first = get_param(sys,'Created');
      | first = first(end-3:end);  %year is last four digits
      | 
      | last = get_param(sys,'LastModifiedDate');
      | if isempty(last)
      |     last = datestr(now,'yyyy');
      | else
      |     last = last(end-3:end);
      | end
      | 
      | if strcmp(first,last)
      |     fprintf('%s -- Copyright %s Nexteer',NxtrConf,first)
      | else
      |     fprintf('%s -- %s%s- %s Nexteer',NxtrConf,char(169),first,last)
      | end
  Ena_FALSE : Constant  RequirementInfo="{'linktype_rmi_doors' '00007fee (/E-STEER Core/SubSystem Specifications/Application Functions/SF004B Assist Summation and Limiting- Current)' '#SF004B_291' 'true' 'REQ:  SF004B_291' '' } %GIDa_53947e4f_d786_4f66_b678_e98c20b24129"  Value=false  OutDataTypeStr=boolean
  Enumerated Constant1 : simulink/Sources/Enumerated Constant  RequirementInfo="{'linktype_rmi_doors' '00007fee (/E-STEER Core/SubSystem Specifications/Application Functions/SF004B Assist Summation and Limiting- Current)' '#SF004B_243' 'true' 'REQ:  SF004B_243' '' } %GIDa_03d8eb68_7ac8_4e07_aa9f_32adb233e68f"  OutDataTypeStr=Enum: NtcNr1  Value=NtcNr1.NTCNR_0X0C4  SampleTime=inf
  Enumerated Constant2 : simulink/Sources/Enumerated Constant  RequirementInfo="{'linktype_rmi_doors' '00007fee (/E-STEER Core/SubSystem Specifications/Application Functions/SF004B Assist Summation and Limiting- Current)' '#SF004B_243' 'true' 'REQ:  SF004B_243' '' } %GIDa_7fc9015b_e364_4d1e_8eea_7193020fb723"  OutDataTypeStr=Enum: NtcSts1  Value=NtcSts1.NTCSTS_PREFAILD  SampleTime=inf
  Enumerated Constant4 : simulink/Sources/Enumerated Constant  RequirementInfo="{'linktype_rmi_doors' '00007fee (/E-STEER Core/SubSystem Specifications/Application Functions/SF004B Assist Summation and Limiting- Current)' '#SF004B_243' 'true' 'REQ:  SF004B_243' '' } %GIDa_bfed8754_6476_47b4_95e4_88ba466e576f"  OutDataTypeStr=Enum: NtcSts1  Value=NtcSts1.NTCSTS_PREPASSD  SampleTime=inf
  Enumerated Constant6 : simulink/Sources/Enumerated Constant  RequirementInfo="{'linktype_rmi_doors' '00007fee (/E-STEER Core/SubSystem Specifications/Application Functions/SF004B Assist Summation and Limiting- Current)' '#SF004B_243' 'true' 'REQ:  SF004B_243' '' } %GIDa_59800a20_b7df_4cb1_bc83_58e7943c9eb7"  OutDataTypeStr=Enum: NtcNr1  Value=NtcNr1.NTCNR_0X0C4  SampleTime=inf
  If2 : If  RequirementInfo="{'linktype_rmi_doors' '00007fee (/E-STEER Core/SubSystem Specifications/Application Functions/SF004B Assist Summation and Limiting- Current)' '#SF004B_243' 'true' 'REQ:  SF004B_243' '' } %GIDa_5db6f1d7_eb54_4ae2_be13_2ab927c6e953"  IfExpression=~u1
  Logical Operator2 : Logic  RequirementInfo="{'linktype_rmi_doors' '00007fee (/E-STEER Core/SubSystem Specifications/Application Functions/SF004B Assist Summation and Limiting- Current)' '#SF004B_243' 'true' 'REQ:  SF004B_243' '' } %GIDa_17204dbd_746f_4295_b165_30eaf18d39eb"  Operator=OR  AllPortsSameDT=off  OutDataTypeStr=boolean
  ManTqCmdZero : Constant  RequirementInfo="{'linktype_rmi_doors' '00007fee (/E-STEER Core/SubSystem Specifications/Application Functions/SF004B Assist Summation and Limiting- Current)' '#SF004B_290' 'true' 'REQ:  SF004B_290' '' } %GIDa_dd78220a_46f6_43c1_a166_2d84650302c6"  Value=MOTTQZERO_MOTNWTMTR_F32
  Relational Operator2 : RelationalOperator  RequirementInfo="{'linktype_rmi_doors' '00007fee (/E-STEER Core/SubSystem Specifications/Application Functions/SF004B Assist Summation and Limiting- Current)' '#SF004B_243' 'true' 'REQ:  SF004B_243' '' } %GIDa_22a0ed4e_e74a_43b7_9e8c_7d4c52cdfc10"  Operator=>  OutDataTypeStr=boolean
  SetNtcSts1 : Subsystem  RequirementInfo="{'linktype_rmi_doors' '00007fee (/E-STEER Core/SubSystem Specifications/Application Functions/SF004B Assist Summation and Limiting- Current)' '#SF004B_243' 'true' 'REQ:  SF004B_243' '' } %GIDa_af2c5d98_11b5_417a_be68_dbcb77b832ee"  mask(SetNTC){}
      mask help: SetNTC library block
  SetNtcSts2 : Subsystem  RequirementInfo="{'linktype_rmi_doors' '00007fee (/E-STEER Core/SubSystem Specifications/Application Functions/SF004B Assist Summation and Limiting- Current)' '#SF004B_243' 'true' 'REQ:  SF004B_243' '' } %GIDa_69402f2f_9b2f_4d96_9c27_f1aa157b908c"  mask(SetNTC){}
      mask help: SetNTC library block
  ManTqCmdEnaOut : Outport  RequirementInfo="{'linktype_rmi_doors' '00007fee (/E-STEER Core/SubSystem Specifications/Application Functions/SF004B Assist Summation and Limiting- Current)' '#SF004B_291' 'true' 'REQ:  SF004B_291' '' } %GIDa_88ec41a0_fd78_45e7_a4c2_2953d2f1273a"
  ManTqCmdOut : Outport  RequirementInfo="{'linktype_rmi_doors' '00007fee (/E-STEER Core/SubSystem Specifications/Application Functions/SF004B Assist Summation and Limiting- Current)' '#SF004B_290' 'true' 'REQ:  SF004B_290' '' } %GIDa_779fe8cb_154f_4893_925f_561d4f3b3ad1"  Port=2
  wires:
  Constant2/1 -> Relational Operator2/2
  Abslt_f32_f1/1 -> Relational Operator2/1
  PinionCentrLrnCmd/1 -> Abslt_f32_f1/1
  PinionCentrLrnEna/1 -> Logical Operator2/1
  Relational Operator2/1 -> Logical Operator2/2
  Ena_FALSE/1 -> ManTqCmdEnaOut/1
  ManTqCmdZero/1 -> ManTqCmdOut/1
  If2/1 -> SetNtcSts1/Action
  Enumerated Constant6/1 -> SetNtcSts1/1(NtcNr)
  Constant6/1 -> SetNtcSts1/2(NtcStInfo)
  Enumerated Constant4/1 -> SetNtcSts1/3(NtcSts)
  Constant5/1 -> SetNtcSts1/4(DebStep)
  Enumerated Constant1/1 -> SetNtcSts2/1(NtcNr)
  Constant4/1 -> SetNtcSts2/2(NtcStInfo)
  Enumerated Constant2/1 -> SetNtcSts2/3(NtcSts)
  Constant1/1 -> SetNtcSts2/4(DebStep)
  If2/2 -> SetNtcSts2/Action
  Logical Operator2/1 -> If2/1

== system SF004B_AssiSumLim/AssiSumLim/SetManTqCmd/ELSE/CopyRight2 ==

== system SF004B_AssiSumLim/AssiSumLim/SetManTqCmd/THEN/CopyRight2 ==

== system SF004B_AssiSumLim/AssiSumLim/SetManTqCmd/THEN/If Action Subsystem ==
  In1 : Inport
  In2 : Inport  Port=2
  In3 : Inport  Port=3
  Action Port : ActionPort  ActionType=then
  CopyRight2 : Subsystem  Description=|  mask(Copyright Information){none=on}
      | Copyright info block.                                               
      |                                                                     
      | Place copyright information at the top of every subsystem in design.
      mask prompts: none "No parameters"
      mask help: Place copyright information at the top of every subsystem in design.
      mask Display:
      | NxtrConf = 'Nexteer Confidential';
      | 
      | sys = bdroot; %handle for the current model ("system")
      | first = get_param(sys,'Created');
      | first = first(end-3:end);  %year is last four digits
      | 
      | last = get_param(sys,'LastModifiedDate');
      | if isempty(last)
      |     last = datestr(now,'yyyy');
      | else
      |     last = last(end-3:end);
      | end
      | 
      | if strcmp(first,last)
      |     fprintf('%s -- Copyright %s Nexteer',NxtrConf,first)
      | else
      |     fprintf('%s -- %s%s- %s Nexteer',NxtrConf,char(169),first,last)
      | end
  Out1 : Outport
  Out2 : Outport  Port=2
  Out3 : Outport  Port=3
  wires:
  In1/1 -> Out1/1
  In2/1 -> Out2/1
  In3/1 -> Out3/1
